simulink model "complete_controller_unorganized"  (R2023a)
settings: Solver=FixedStepAuto  StartTime=0.0  StopTime=inf  FixedStep=0.01  RelTol=1e-3
model workspace (MAT data in the model file):
  SL_ROS_VariableLengthArrays_MaxSizes : object (value not decoded)
undefined symbols (not defined in the file): angular, Btrigger_boost, DAapply_nudges, DAdesired_pose, DAff_body_force, DAsolver_weights, Djoy_R_X, Dreverse_throttle, Dthrottle, Iangular_mode, Ilinear_mode, linear
libraries: ros2lib x78
(part 3 of 3)

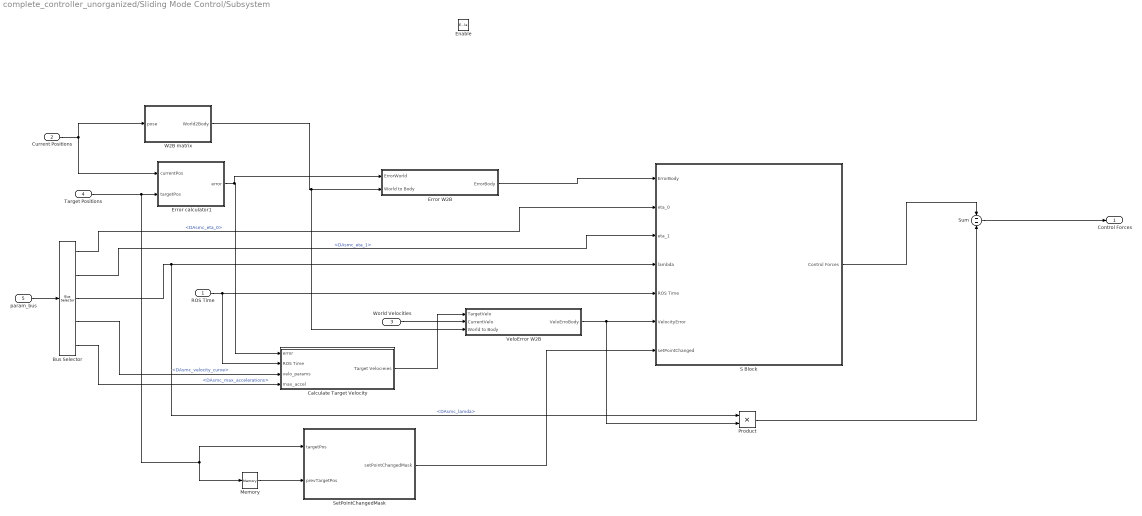
== system complete_controller_unorganized/Sliding Mode Control/Subsystem ==
  ROS Time : Inport
  Current Positions : Inport  Port=2
  World Velocities : Inport  Port=3
  Target Positions : Inport  Port=4
  param_bus : Inport  Port=5
  Enable : EnablePort
  Bus Selector : BusSelector  OutputSignals=DAsmc_eta_0,DAsmc_eta_1,DAsmc_lamda,DAsmc_velocity_curve,DAsmc_max_accelerations
  Calculate Target Velocity : Subsystem
  Error W2B : Subsystem
  Error calculator1 : MATLAB Function  TreatAsAtomicUnit=on
  Memory : Memory
  Product : Product
  S Block : Subsystem
  SetPointChangedMask : MATLAB Function  TreatAsAtomicUnit=on
  Sum : Sum  Inputs=--
  VeloError W2B : Subsystem
  W2B matrix : MATLAB Function  TreatAsAtomicUnit=on
  Control Forces : Outport
  wires:
  Target Positions/1 -> Memory/1, SetPointChangedMask/1(targetPos), Error calculator1/2(targetPos)
  Current Positions/1 -> W2B matrix/1(pose), Error calculator1/1(currentPos)
  ROS Time/1 -> Calculate Target Velocity/2(ROS Time), S Block/5(ROS Time)
  Error calculator1/1(error) -> Error W2B/1(ErrorWorld), Calculate Target Velocity/1(error)
  param_bus/1 -> Bus Selector/1
  Bus Selector/5 -> Calculate Target Velocity/4(max_accel)  "<DAsmc_max_accelerations>"
  Bus Selector/4 -> Calculate Target Velocity/3(velo_params)  "<DAsmc_velocity_curve>"
  Bus Selector/2 -> S Block/3(eta_1)  "<DAsmc_eta_1>"
  Bus Selector/1 -> S Block/2(eta_0)  "<DAsmc_eta_0>"
  Bus Selector/3 -> S Block/4(lambda), Product/1  "<DAsmc_lamda>"
  World Velocities/1 -> VeloError W2B/2(CurrentVelo)
  Calculate Target Velocity/1(Target Velocieies) -> VeloError W2B/1(TargetVelo)
  Error W2B/1(ErrorBody) -> S Block/1(ErrorBody)
  W2B matrix/1(World2Body) -> VeloError W2B/3(World to Body), Error W2B/2(World to Body)
  VeloError W2B/1(VeloErroBody) -> Product/2, S Block/6(VelocityError)
  Memory/1 -> SetPointChangedMask/2(prevTargetPos)
  SetPointChangedMask/1(setPointChangedMask) -> S Block/7(setPointChanged)
  S Block/1(Control Forces) -> Sum/1
  Sum/1 -> Control Forces/1
  Product/1 -> Sum/2

== system complete_controller_unorganized/PID Control2/Enabled Subsystem/Error W2B ==
  ErrorWorld : Inport
  World to Body : Inport  Port=2
  Demux4 : Demux  Outputs=6
  MatrixMultiply8 : Product  Multiplication=Matrix(*)
  Mux16 : Mux  Inputs=3
  Mux17 : Mux  Inputs=3
  Mux18 : Mux  Inputs=2
  ErrorBody : Outport
  wires:
  Demux4/2 -> Mux16/2
  Demux4/4 -> Mux17/1
  Mux16/1 -> MatrixMultiply8/2
  Demux4/6 -> Mux17/3
  Demux4/1 -> Mux16/1
  Demux4/5 -> Mux17/2
  Mux17/1 -> Mux18/2
  ErrorWorld/1 -> Demux4/1
  Demux4/3 -> Mux16/3
  MatrixMultiply8/1 -> Mux18/1
  Mux18/1 -> ErrorBody/1
  World to Body/1 -> MatrixMultiply8/1

== system complete_controller_unorganized/PID Control2/Enabled Subsystem/Velocities W2B ==
  Velocities World : Inport
  World to Body : Inport  Port=2
  Demux4 : Demux  Outputs=6
  MatrixMultiply8 : Product  Multiplication=Matrix(*)
  Mux16 : Mux  Inputs=3
  Mux17 : Mux  Inputs=3
  Mux18 : Mux  Inputs=2
  Velocities Body : Outport
  wires:
  Demux4/2 -> Mux16/2
  Demux4/4 -> Mux17/1
  Mux16/1 -> MatrixMultiply8/2
  Demux4/6 -> Mux17/3
  Demux4/1 -> Mux16/1
  Demux4/5 -> Mux17/2
  Mux17/1 -> Mux18/2
  Velocities World/1 -> Demux4/1
  Demux4/3 -> Mux16/3
  MatrixMultiply8/1 -> Mux18/1
  Mux18/1 -> Velocities Body/1
  World to Body/1 -> MatrixMultiply8/1

== system complete_controller_unorganized/PID Control2/Enabled Subsystem/iGains W2B ==
  iGains World : Inport
  World to Body : Inport  Port=2
  Demux4 : Demux  Outputs=6
  MatrixMultiply8 : Product  Multiplication=Matrix(*)
  Mux16 : Mux  Inputs=3
  Mux17 : Mux  Inputs=3
  Mux18 : Mux  Inputs=2
  iGains Body : Outport
  wires:
  Demux4/2 -> Mux16/2
  Demux4/4 -> Mux17/1
  Mux16/1 -> MatrixMultiply8/2
  Demux4/6 -> Mux17/3
  Demux4/1 -> Mux16/1
  Demux4/5 -> Mux17/2
  Mux17/1 -> Mux18/2
  iGains World/1 -> Demux4/1
  Demux4/3 -> Mux16/3
  MatrixMultiply8/1 -> Mux18/1
  Mux18/1 -> iGains Body/1
  World to Body/1 -> MatrixMultiply8/1

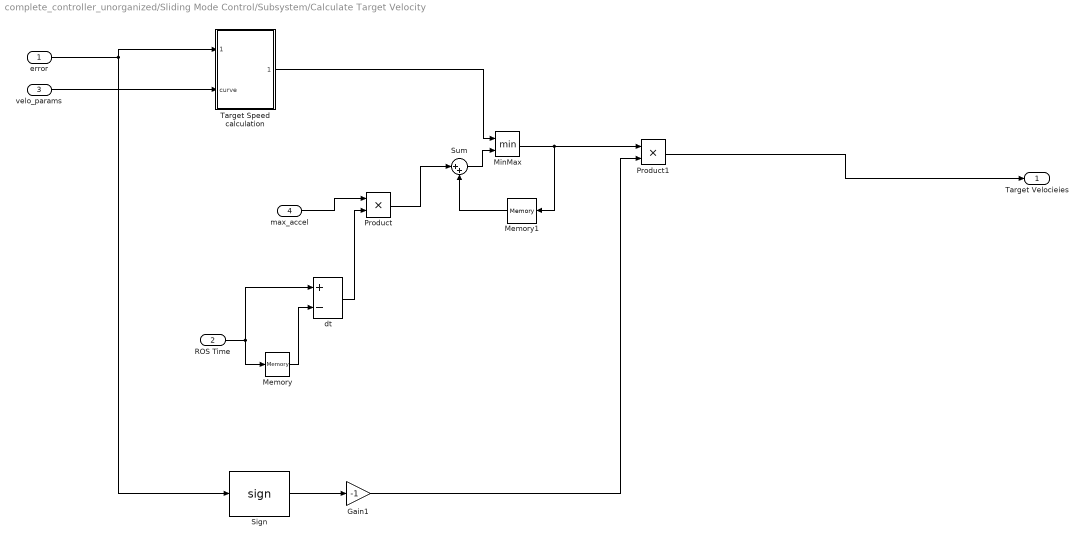
== system complete_controller_unorganized/Sliding Mode Control/Subsystem/Calculate Target Velocity ==
  error : Inport
  ROS Time : Inport  Port=2
  velo_params : Inport  Port=3
  max_accel : Inport  Port=4
  Gain1 : Gain  Gain=-1
  Memory : Memory
  Memory1 : Memory
  MinMax : MinMax  Inputs=2
  Product : Product
  Product1 : Product
  Sign : Signum
  Sum : Sum  Inputs=|++
  Target Speed calculation : MATLAB Function  TreatAsAtomicUnit=on
  dt : Sum  Inputs=+-
  Target Velocieies : Outport
  wires:
  error/1 -> Sign/1, Target Speed calculation/1(posError)
  ROS Time/1 -> Memory/1, dt/1
  Memory/1 -> dt/2
  velo_params/1 -> Target Speed calculation/2(curve)
  Target Speed calculation/1(targetSpeed) -> MinMax/1
  max_accel/1 -> Product/1
  dt/1 -> Product/2
  Product/1 -> Sum/1
  MinMax/1 -> Product1/1, Memory1/1
  Memory1/1 -> Sum/2
  Sum/1 -> MinMax/2
  Sign/1 -> Gain1/1
  Product1/1 -> Target Velocieies/1
  Gain1/1 -> Product1/2

== system complete_controller_unorganized/Sliding Mode Control/Subsystem/Error W2B ==
  ErrorWorld : Inport
  World to Body : Inport  Port=2
  Demux4 : Demux  Outputs=6
  MatrixMultiply8 : Product  Multiplication=Matrix(*)
  Mux16 : Mux  Inputs=3
  Mux17 : Mux  Inputs=3
  Mux18 : Mux  Inputs=2
  ErrorBody : Outport
  wires:
  Demux4/2 -> Mux16/2
  Demux4/4 -> Mux17/1
  Mux16/1 -> MatrixMultiply8/2
  Demux4/6 -> Mux17/3
  Demux4/1 -> Mux16/1
  Demux4/5 -> Mux17/2
  Mux17/1 -> Mux18/2
  ErrorWorld/1 -> Demux4/1
  Demux4/3 -> Mux16/3
  MatrixMultiply8/1 -> Mux18/1
  Mux18/1 -> ErrorBody/1
  World to Body/1 -> MatrixMultiply8/1

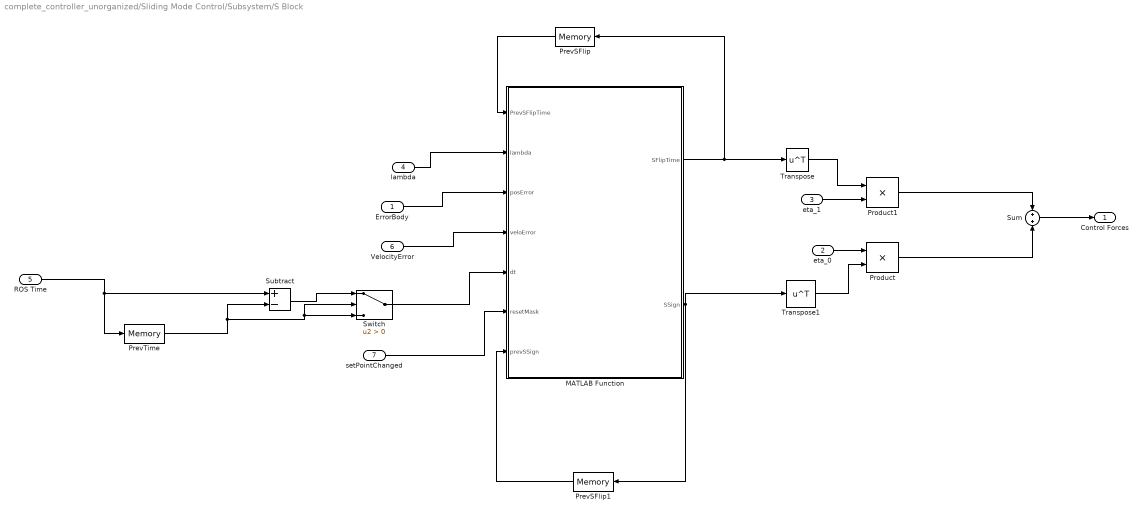
== system complete_controller_unorganized/Sliding Mode Control/Subsystem/S Block ==
  ErrorBody : Inport
  eta_0 : Inport  Port=2
  eta_1 : Inport  Port=3
  lambda : Inport  Port=4
  ROS Time : Inport  Port=5
  VelocityError : Inport  Port=6
  setPointChanged : Inport  Port=7
  MATLAB Function : MATLAB Function  TreatAsAtomicUnit=on
  PrevSFlip : Memory  InitialCondition=[0;0;0;0;0;0]
  PrevSFlip1 : Memory  InitialCondition=[0;0;0;0;0;0]
  PrevTime : Memory
  Product : Product
  Product1 : Product
  Subtract : Sum  Inputs=+-
  Sum : Sum
  Switch : Switch  Criteria=u2 > Threshold  SaturateOnIntegerOverflow=off  InputSameDT=off
  Transpose : Math  Operator=transpose  OutputSignalType=real
  Transpose1 : Math  Operator=transpose  OutputSignalType=real
  Control Forces : Outport
  wires:
  eta_0/1 -> Product/1
  MATLAB Function/2(SSign) -> PrevSFlip1/1, Transpose1/1
  eta_1/1 -> Product1/2
  MATLAB Function/1(SFlipTime) -> Transpose/1, PrevSFlip/1
  Product/1 -> Sum/2
  Sum/1 -> Control Forces/1
  lambda/1 -> MATLAB Function/2(lambda)
  ErrorBody/1 -> MATLAB Function/3(posError)
  VelocityError/1 -> MATLAB Function/4(veloError)
  PrevSFlip/1 -> MATLAB Function/1(PrevSFlipTime)
  ROS Time/1 -> PrevTime/1, Subtract/1
  Subtract/1 -> Switch/1
  Switch/1 -> MATLAB Function/5(dt)
  PrevTime/1 -> Switch/3, Switch/2, Subtract/2
  setPointChanged/1 -> MATLAB Function/6(resetMask)
  Transpose/1 -> Product1/1
  PrevSFlip1/1 -> MATLAB Function/7(prevSSign)
  Transpose1/1 -> Product/2
  Product1/1 -> Sum/1

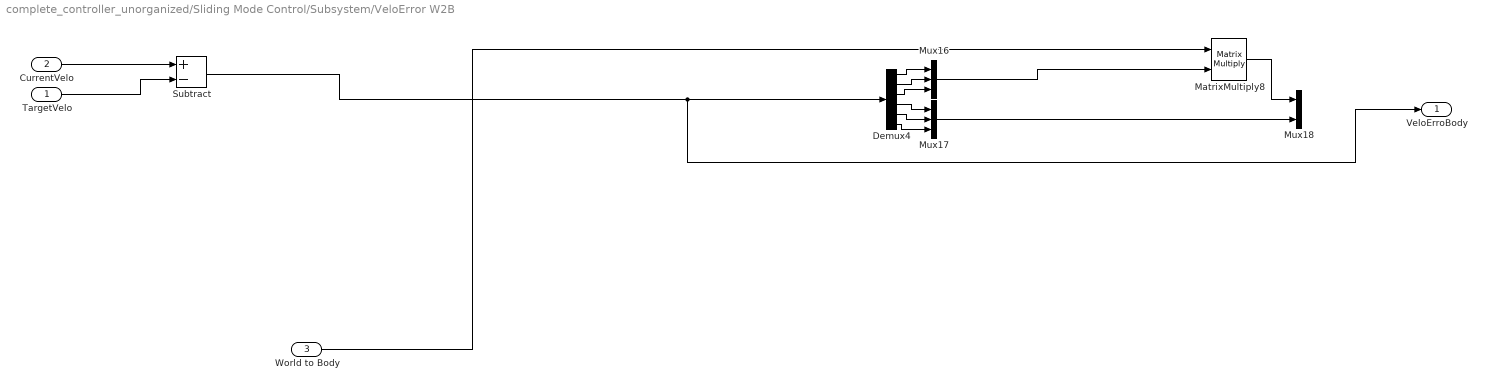
== system complete_controller_unorganized/Sliding Mode Control/Subsystem/VeloError W2B ==
  TargetVelo : Inport
  CurrentVelo : Inport  Port=2
  World to Body : Inport  Port=3
  Demux4 : Demux  Outputs=6
  MatrixMultiply8 : Product  Multiplication=Matrix(*)
  Mux16 : Mux  Inputs=3
  Mux17 : Mux  Inputs=3
  Mux18 : Mux  Inputs=2
  Subtract : Sum  Inputs=+-
  VeloErroBody : Outport
  wires:
  Demux4/2 -> Mux16/2
  Demux4/4 -> Mux17/1
  Mux16/1 -> MatrixMultiply8/2
  Demux4/6 -> Mux17/3
  Demux4/1 -> Mux16/1
  Demux4/5 -> Mux17/2
  Mux17/1 -> Mux18/2
  TargetVelo/1 -> Subtract/2
  Demux4/3 -> Mux16/3
  MatrixMultiply8/1 -> Mux18/1
  World to Body/1 -> MatrixMultiply8/1
  CurrentVelo/1 -> Subtract/1
  Subtract/1 -> VeloErroBody/1, Demux4/1

== matlab function complete_controller_unorganized/PID Control2/MATLAB Function ==
  data: pose input; World2Body output
function World2Body= fcn(pose)

poseQuat = [pose(7), pose(4), pose(5), pose(6)];

World2Body = transpose(quat2rotm(poseQuat));

== matlab function complete_controller_unorganized/Sliding Mode Control/Subsystem/Calculate Target Velocity/Target Speed calculation ==
  data: posError input; targetSpeed output; curve input
function targetSpeed = fcn(posError, curve)

targetSpeed = zeros(1,6);
if(~length(curve) == 12)
    %params have not yet been assigned / assgined incorrectly
    fprintf("Velo curves not initilized properly! /n");
    return
end

curve = reshape(curve, 2, 6);

%param(1,x) = max control value
%param(2,x) = the error where max control is reached
%velocity curves = param(1,x) * (-cos(error * pi / (2 * param(2,x)))^1/2 + 1)
for i=1:6
    if(posError(i) == 0 || curve(2,i) == 0)
        targetSpeed(i) = 0;
    else
        if(abs(posError(i)) > curve(2,i))
            posError(i) = curve(2,i)*sign(posError(i));
        end
        
        targetSpeed(i) = curve(1, i) * (1-(abs(cos(posError(i)*pi/(2*curve(2,i))))^(1/2)));
       
    end
end

== matlab function complete_controller_unorganized/Sliding Mode Control/Subsystem/Error calculator1 ==
  data: currentPos input; targetPos input; error output
function error = fcn(currentPos, targetPos)

error = zeros(1,6);

%World Frame linear error
eWorld = zeros(1,3);

eWorld(1) = currentPos(1) - targetPos(1);
eWorld(2) = currentPos(2) - targetPos(2);
eWorld(3) = currentPos(3) - targetPos(3);

%Quaternion that represents position
currentQuat = [currentPos(7), currentPos(4), currentPos(5), currentPos(6)];

%make it a unit quaternion
unitQuat = currentQuat ./ norm(currentQuat);

%quaternion that we want to be at
setQuat = [targetPos(7), -targetPos(4), -targetPos(5), -targetPos(6)];

uSetQuat = setQuat ./ norm(setQuat);

%multiply the inverse of the unit quat by the set quat to get an error
eQuat = quatmultiply(uSetQuat, conj(unitQuat));
if(eQuat(1) < 0) 
    eQuat = -eQuat;
end

%total rotation angle
w = max(min(eQuat(1),1),-1);
theta = 2 * acos(w);
%sin(theta/2)
s = sqrt(max(1 - w^2,0));
%rotation axis and rotation vector
if s < 1e-6
   eRot = [0 0 0];
else
   axis = eQuat(2:4) / s;
   eRot = theta * axis;
end

theta_mag = norm(eRot);
if theta_mag < 1e-9
   axisError = [0 0 0];
else
   axisError = (sin(theta_mag/2)/theta_mag) * eRot;
end



error(1) = eWorld(1);
error(2) = eWorld(2);
error(3) = eWorld(3);
error(4) = axisError(1);
error(5) = axisError(2);
error(6) = axisError(3);

fprintf("Error:")
disp(error)
end




% error(4) = eVector(1);
% error(5) = eVector(2);
% error(6) = eVector(3);

% function normalizedError = fcn(currentPosition, currentSetPoint)
% 
% normalized = zeros(1,6);
% 
% normalized(1) = -(currentPosition(1) - currentSetPoint(1));
% normalized(2) = -(currentPosition(2) - currentSetPoint(2));
% normalized(3) = -(currentPosition(3) - currentSetPoint(3));
% 
% W2B = [currentPosition(4), currentPosition(5), currentPosition(6), currentPosition(7)];
% setQuat = [currentSetPoint(4), -currentSetPoint(5), -currentSetPoint(6), -currentSetPoint(7)];
% 
% 
% %Talos Heading in Body Frame
% Tbody = [1,0,0,0];
% 
% %Transform from Body 2 World
% B2W = [W2B(1), -W2B(2), -W2B(3), -W2B(4)] / (norm(W2B) ^ 2);
% 
% %Talos Heading in World Frame
% TWorld = quatmultiply(Tbody, B2W);
% 
% %Talos Heading in World Frame Conjugate
% TWorldI = [TWorld(1), -TWorld(2), -TWorld(3), -TWorld(4)];
% 
% %Current Yaw Error
% eQuat = quatmultiply(setQuat, TWorldI);
% 
% % %axis Error
% axisError = [eQuat(2), eQuat(3), eQuat(4)];
% if(eQuat(1) < 0)
%     axisError = -axisError;
% end
% 
% 
% normalized(4) = axisError(1);
% normalized(5) = axisError(2);
% normalized(6) = axisError(3);
% 
% normalizedError = normalized;

== matlab function complete_controller_unorganized/Sliding Mode Control/Subsystem/S Block/MATLAB Function ==
  data: PrevSFlipTime input; lambda input; posError input; veloError input; dt input; SFlipTime output; resetMask input; SSign output; prevSSign input
function [SFlipTime, SSign] = fcn(PrevSFlipTime, lambda, posError, veloError, dt, resetMask, prevSSign)


SFlipTime = PrevSFlipTime;
SSign = zeros(6,1);

S = posError + veloError' .* lambda';

for i=1:6
    SSign(i) = sign(S(i));
end


for i=1:6
    if(~resetMask(i))
        if(prevSSign(i) == SSign(i))
            SFlipTime(i) = SFlipTime(i) + SSign(i) * dt;
        else
            SFlipTime(i) = SSign(i) * dt;
        end
    else
        SFlipTime(i) = 0;
    end
end

== matlab function complete_controller_unorganized/com learner ==
  data: average_error input; new_state output; previous_adjustment_average_error input; previous_state input; previous_rewards input; resolution input; previous_application input; total_time input; eval_time input; rewards output; application output; latest_adjustment_average_error output; last_applied output; previous_last_applied input; reset_accumulator output
function [new_state, rewards, application, latest_adjustment_average_error, last_applied, reset_accumulator] = com_leaner(average_error, previous_adjustment_average_error, previous_state, previous_rewards, resolution, previous_application, total_time, eval_time, previous_last_applied)

error_sum = sum(average_error(1:3));

latest_adjustment_average_error = previous_adjustment_average_error;
application = previous_application;
rewards = previous_rewards;
new_state = previous_state;
last_applied = previous_last_applied;
reset_accumulator = false;

if(total_time > eval_time)
    %time to apply com
    if(new_state == 0)
        %set the baseline
        latest_adjustment_average_error = error_sum;

        %increment the first application
        application = application + [resolution, 0, 0]';
        last_applied = 1;

        %increment the state
        new_state = new_state + 1;
    elseif(new_state == 1)
        %set the reward for this adjustment
        rewards(1) = latest_adjustment_average_error - error_sum;

        %increment the first application
        application = application + [-2 * resolution, 0, 0]';
        last_applied = -1;


        %increment the state
        new_state = new_state + 1;
    elseif(new_state == 2)
        %set the reward for this adjustment
        rewards(2) = latest_adjustment_average_error - error_sum;

        %increment the first application
        application = application + [resolution, resolution, 0]';
        last_applied = 2;


        %increment the state
        new_state = new_state + 1;
    elseif(new_state == 3)
        %set the reward for this adjustment
        rewards(3) = latest_adjustment_average_error - error_sum;

        %increment the first application
        application = application + [0, -2*resolution, 0]';
        last_applied = -2;


        %increment the state
        new_state = new_state + 1;
   elseif(new_state == 4)
        %set the reward for this adjustment
        rewards(4) = latest_adjustment_average_error - error_sum;

        %increment the first application
        application = application + [0, resolution, resolution]';
        last_applied = 3;


        %increment the state
        new_state = new_state + 1;
    elseif(new_state == 5)
        %set the reward for this adjustment
        rewards(5) = latest_adjustment_average_error - error_sum;

        %increment the first application
        application = [0, 0, -2*resolution]';
        last_applied = -3;


        %increment the state
        new_state = new_state + 1;
    elseif(new_state == 6)
        application = application + [0, 0, resolution]';

        %set the reward for this adjustment
        rewards(6) = latest_adjustment_average_error - error_sum;

        %apply the best option
        [~, index] = max(rewards);
        apply_index = ceil(index / 2);
        apply_sign = (1 - 2 * mod(index, 2));
        application(apply_index) = application(apply_index) + resolution * apply_sign;
        last_applied = apply_sign * apply_index;

        %increment the state
        new_state = new_state + 1;
    elseif(new_state == 7)
        %update the reward for the previously applied

        if(latest_adjustment_average_error - error_sum < 0)
            %undo the last action if it was bad
            application(abs(last_applied)) = application(abs(last_applied)) - resolution * sign(last_applied);
        end

        rewards((abs(last_applied) * 2) + (-sign(last_applied) + 1) / 2 - 1) = latest_adjustment_average_error - error_sum;
        latest_adjustment_average_error = error_sum;

        if(max(rewards) < 0)
            new_state = 0;
        else
            %apply the best option
            [~, index] = max(rewards);
            apply_index = ceil(index / 2);
            apply_sign = -(1 - 2 * mod(index, 2));
            application(apply_index) = application(apply_index) + resolution * apply_sign;
            last_applied = apply_sign * apply_index;
        end

    end

    reset_accumulator = true;
   
end

== matlab function complete_controller_unorganized/PID Control2/Enabled Subsystem/Error calculator1 ==
  data: currentPos input; targetPos input; error output
function error = fcn(currentPos, targetPos)

error = zeros(1,6);

%World Frame linear error
eWorld = zeros(1,3);

eWorld(1) = currentPos(1) - targetPos(1);
eWorld(2) = currentPos(2) - targetPos(2);
eWorld(3) = currentPos(3) - targetPos(3);

%Quaternion that represents position
currentQuat = [currentPos(7), currentPos(4), currentPos(5), currentPos(6)];

%make it a unit quaternion
unitQuat = currentQuat ./ norm(currentQuat);

%quaternion that we want to be at
setQuat = [targetPos(7), -targetPos(4), -targetPos(5), -targetPos(6)];

uSetQuat = setQuat ./ norm(setQuat);

%multiply the unit setQuat by the conjugate of the unit quaternion
eQuat = quatmultiply(uSetQuat, conj(unitQuat));
if(eQuat(1) < 0) 
    eQuat = -eQuat;
end

%total rotation angle
w = max(min(eQuat(1),1),-1);
theta = 2 * acos(w);
%sin(theta/2)
s = sqrt(max(1 - w^2,0));
%rotation axis and rotation vector
if s < 1e-6
   eRot = [0 0 0];
else
   axis = eQuat(2:4) / s;
   eRot = theta * axis;
end

theta_mag = norm(eRot);
if theta_mag < 1e-9
   axisError = [0 0 0];
else
   axisError = (sin(theta_mag/2)/theta_mag) * eRot;
end



error(1) = eWorld(1);
error(2) = eWorld(2);
error(3) = eWorld(3);
error(4) = axisError(1);
error(5) = axisError(2);
error(6) = axisError(3);
end




% error(4) = eVector(1);
% error(5) = eVector(2);
% error(6) = eVector(3);

% function normalizedError = fcn(currentPosition, currentSetPoint)
% 
% normalized = zeros(1,6);
% 
% normalized(1) = -(currentPosition(1) - currentSetPoint(1));
% normalized(2) = -(currentPosition(2) - currentSetPoint(2));
% normalized(3) = -(currentPosition(3) - currentSetPoint(3));
% 
% W2B = [currentPosition(4), currentPosition(5), currentPosition(6), currentPosition(7)];
% setQuat = [currentSetPoint(4), -currentSetPoint(5), -currentSetPoint(6), -currentSetPoint(7)];
% 
% 
% %Talos Heading in Body Frame
% Tbody = [1,0,0,0];
% 
% %Transform from Body 2 World
% B2W = [W2B(1), -W2B(2), -W2B(3), -W2B(4)] / (norm(W2B) ^ 2);
% 
% %Talos Heading in World Frame
% TWorld = quatmultiply(Tbody, B2W);
% 
% %Talos Heading in World Frame Conjugate
% TWorldI = [TWorld(1), -TWorld(2), -TWorld(3), -TWorld(4)];
% 
% %Current Yaw Error
% eQuat = quatmultiply(setQuat, TWorldI);
% 
% % %axis Error
% axisError = [eQuat(2), eQuat(3), eQuat(4)];
% if(eQuat(1) < 0)
%     axisError = -axisError;
% end
% 
% 
% normalized(4) = axisError(1);
% normalized(5) = axisError(2);
% normalized(6) = axisError(3);
% 
% normalizedError = normalized;

== matlab function complete_controller_unorganized/Sliding Mode Control/Subsystem/SetPointChangedMask ==
  data: targetPos input; setPointChangedMask output; prevTargetPos input
function setPointChangedMask = fcn(targetPos, prevTargetPos)

setPointChangedMask = zeros(6,1);
for i=1:6
    if(targetPos(i) ~= prevTargetPos(i))
        setPointChangedMask(i) = 1;
    else 
        setPointChangedMask(i) = 0;
    end
end

== matlab function complete_controller_unorganized/Sliding Mode Control/Subsystem/W2B matrix ==
  data: pose input; World2Body output
function World2Body= fcn(pose)

poseQuat = [pose(7), pose(4), pose(5), pose(6)];

World2Body = transpose(quat2rotm(poseQuat));

== matlab function complete_controller_unorganized/PID Control2/Enabled Subsystem/MATLAB Function ==
  data: error input; haveGainsChanged input; reset input; currentTime input; prevTime input; prevSum input; sumOfError output
function sumOfError = fcn(error, haveGainsChanged, reset, currentTime, prevTime, prevSum)

dt = 0;
if(prevTime == 0)
    sumOfError = zeros(1,6);
    return
else
    dt = currentTime-prevTime;
end

if(reset || haveGainsChanged)
    sumOfError = zeros(1,6);
    return
end

sumOfError = zeros(1,6);

%check each degree of freedom
for i = 1:6
    sumOfError(i) = (error(i)) * dt + prevSum(i);

    %reset if nan
    if(isnan(error(i)))
        sumOfError(i) = 0;
    end

end

end

== matlab function complete_controller_unorganized/Control Mask Management/MATLAB Function ==
  data: mask_changed output; SMC_Control input; active_control output; PID_Control input; Teleop_Control input; Stunt_Control input; mask input; current_mask output; previous_mask input
function [mask_changed, active_control, current_mask] = fcn(SMC_Control, PID_Control, Teleop_Control, Stunt_Control, mask, previous_mask)

%mux together both the SMC and PID control outputs

active_control = zeros(6,1);

for i=1:6

    if (mask(i) == 2)
        active_control(i) = SMC_Control(i);
    end

    if (mask(i) == 1)
        active_control(i) = PID_Control(i);
    end    
    
    if (mask(i) == 3)
        active_control(i) = Teleop_Control(i);
    end

    if(mask(i) == 4)
        active_control(i) = Stunt_Control(i);
    end

end

mask_changed = 1;
if(isequal(previous_mask, mask))
    mask_changed = 0;
end

current_mask = mask;

== matlab function complete_controller_unorganized/TeleOp/MATLAB Function1 ==
  data: current_body_velocities input; throttle input; reverse input; joy_R_X input; apply_nudge input; teleop_control output; throttle_deadzone input; nudge_forces input; max_steering_angle input; width input; accel_force input; drag_coefficent input; reverse_max_force_multiplier input; boost input
function teleop_control = fcn(current_body_velocities, throttle, reverse, joy_R_X, apply_nudge, throttle_deadzone, nudge_forces, max_steering_angle, width, accel_force, drag_coefficent, reverse_max_force_multiplier, boost)

% @throttle - the percentage of the defined max speed to move forward at -
% scalar
% @brake - the percentage of the breaks to apply
% @throttle_deadzone - the minimum throttle position to move into - scalar
% @apply nudge - if to apply nudge in each dof (x,y,yaw)- 6x1 [contrain to 1, 0, -1]
% @nudge_forces - the force to nudge with in each dof (x,y,yaw) - 6x1
% @joy_L_X - the left joystick x input - scalar
% @max_steering_angle - the maximum simulated steering angle
% @width - robot width - scalar
% @accel force - the force to accelerate with - scalar
% @drag coefficent - the drag coefficent - scalar (N / (m /s) ^2)
% @current_body_velocities - from odom - 6x1
% @boost - the amount to boost the acceleration - scalar


%this should only output non-zero values for x, y and yaw - roll pitch and
%depth are left to PID
teleop_control = zeros(6,1);

%Rocket Leauge -- Sorta Kinda

%if throtlle essentially zero, move into nudge mode
if(abs(throttle) < throttle_deadzone)

    %nudges from yaw come from left joystick
    apply_nudge(6) = joy_R_X; 

    %apply nudge forces
    for i = 1:6

        %either forward backward or not at all
        if(apply_nudge(i) > .5)
            teleop_control(i) = nudge_forces(i);
        elseif (apply_nudge(i) < -.5)
            teleop_control(i) = -1 * nudge_forces(i);
        end
    end

else
    
    %restrict brake values
    throttle = min(max(throttle,0), 1);

    reverse = min(max(reverse, 0), 1) * reverse_max_force_multiplier;

    %factor reverse into throttle
    throttle = throttle - reverse;

    %restrict joystick values
    joy_R_X = min(max(joy_R_X,-1), 1);

    %constrain boost
    boost = max(boost, 1);

    %apply boost
    throttle = throttle * boost;

    %ackermann steering
    %f_outer = k sqrt(v / 2pi * (1 + (w * 2pi * theta / l * 360)))
    %f_inner = k sqrt(v / 2pi * (1 - (w * 2pi * theta / l * 360)))
    %assume L = 2w for car like properties
    %assuming acceleratory force is much less than steady state...

    length = 2*width;

    %I designed this to bypass solver (face smack)
    v_outer = abs(current_body_velocities(1)) / 2 * pi() * (1 + (width * 2 * pi()) * max_steering_angle * abs(joy_R_X) / (length * 360));
    v_inner = abs(current_body_velocities(1)) / 2 * pi() * (1 - (width * 2 * pi()) * max_steering_angle * abs(joy_R_X) / (length * 360));

    %apply drag to get the force on the outer and inner half - I know this
    %isnt exactly how this works
    
    f_outer = drag_coefficent / 2 *  v_outer ^ 2;
    f_inner = drag_coefficent / 2 * v_inner ^ 2;

    %convert out and inner thrusts to wrench approx
    teleop_control(1) = accel_force * throttle;
    teleop_control(6) = abs(f_outer - f_inner) * width * sign(joy_R_X) * sign(throttle);
end

== matlab function complete_controller_unorganized/TeleOp/Handle boost ==
  data: ros_time input; trigger_boost input; boost output; boost_multiplier input; boost_cool_down input; boost_duration input; last_start_time input; start_time output
function [boost, start_time] = fcn(ros_time, trigger_boost,boost_multiplier, boost_cool_down, boost_duration, last_start_time)

%all time in sec

%boost of 1 = no boost

%check if boost is running
if(last_start_time + boost_duration > ros_time)
    boost = boost_multiplier;
    start_time = last_start_time;

    return
end

%check if boost is in cooldown
if(last_start_time + boost_duration + boost_cool_down > ros_time)
    boost = 1;
    start_time = last_start_time;
    return
end

%boost is ready to be restarted
if(trigger_boost)
    start_time = ros_time;
    boost = boost_multiplier;

    return
end

%no boost :(
start_time = last_start_time;
boost = 1;

== matlab function complete_controller_unorganized/Stunt Controller/control_mask_regulator ==
  data: control_mask input; control_mode_mask output; stunt_state input; safe_mode input
function control_mode_mask = fcn(control_mask, stunt_state, safe_mode)

% @ control mask - mask to alter
% @ stunt_state - int 
    % 0 - No Stunt
    % 1 - Summersault
    % 2 - Barrel Rool
% @ safe mode - disable stunt mode (parameter to be changed)

control_mode_mask = [2,2,2,1,1,1];

% the value to configure an axis to stunt mode
stunt_mode_value = 4;

% if summersault requested
if(stunt_state == 1)
    if(~safe_mode)
        %give pitch axis to stunt controller
        control_mode_mask(1) = 0;
        control_mode_mask(2) = 0;
        control_mode_mask(3) = 0;
        control_mode_mask(4) = control_mask(4);
        control_mode_mask(5) = stunt_mode_value;
        control_mode_mask(6) = 0;
    end
end

% if barrel roll requested
if(stunt_state == 2)
    if(~safe_mode)
        %give roll axis to stunt controller
        control_mode_mask(1) = 0;
        control_mode_mask(2) = 0;
        control_mode_mask(3) = 0;
        control_mode_mask(4) = stunt_mode_value;
        control_mode_mask(5) = control_mask(5);
        control_mode_mask(6) = 0;
    end
end

== matlab function complete_controller_unorganized/Stunt Controller/stunt_controller ==
  data: safe_mode input; trigger_stunt_state input; summersault_force input; summersault_run_time input; barrel_roll_force input; barrel_roll_run_time input; ros_time input; current_stunt_start_time input; running_stunt_state input; stunt_active_control output; start_time output; running_state output
function [stunt_active_control, start_time, running_state] = execute_stunt(safe_mode, trigger_stunt_state, summersault_force, summersault_run_time, barrel_roll_force, barrel_roll_run_time, ros_time, current_stunt_start_time, running_stunt_state)

% @ trigger_stunt_state - int 
    % 0 - No Stunt
    % 1 - Summersault
    % 2 - Barrel Rool
% @ running_stunt_state - currently running stunt - int
% @ safe mode - disable stunt mode (parameter to be changed)

stunt_active_control = zeros(6,1);

%if in safe mode return
if(safe_mode)
    start_time = -1;
    running_state = 0;
    return
end

%check for detrigger
if(running_stunt_state == 0)
    %no stunt currently running

    if(trigger_stunt_state == 0)
        %no stunt state being requested

        running_state = 0;
        start_time = -1;

        return
    end
end

%check if summersault is running
if(running_stunt_state == 1)

    % check if time is up
    if(ros_time > current_stunt_start_time + summersault_run_time)
    
        %stop stunt
        start_time = current_stunt_start_time;
        running_state = 0;
        return
    else
        %stunt is running
            
        %apply summer sault force
        stunt_active_control(5) = summersault_force;
        start_time = current_stunt_start_time;
        running_state = running_stunt_state;
        return
    end
end

%check if barrel rolling is running
if(running_stunt_state == 2)

    % check if time is up
    if(ros_time > current_stunt_start_time + barrel_roll_run_time)
    
        %stop stunt
        start_time = current_stunt_start_time;
        running_state = 0;
        return
    else
        %stunt is running
            
        %apply summer sault force
        stunt_active_control(4) = barrel_roll_force;
        start_time = current_stunt_start_time;
        running_state = running_stunt_state;
        return
    end
end

%check for trigger - only if start_time has been reset
if(current_stunt_start_time < 0)
    if(trigger_stunt_state ~= 0)

        %if a stunt has been requested
        running_state = trigger_stunt_state;
        start_time = ros_time;

        %motion begin on next loop
        return

    end

end

start_time = current_stunt_start_time;
running_state = running_stunt_state;
